simulink model "SkywalkerX8_Lateral_Verification"  (R2018a)
settings: Solver=FixedStepAuto  StartTime=0.0  StopTime=10.0  FixedStep=0.001  RelTol=1e-3
settings Model: Creator=David  LastModifiedBy=David
settings DataIOCC: SaveFormat=StructureWithTime
settings OptimizationCC: BlockReduction=off  BufferReuse=off
settings DebuggingCC: AlgebraicLoopMsg=none  UnconnectedInputMsg=none  UnconnectedOutputMsg=none  UnconnectedLineMsg=none

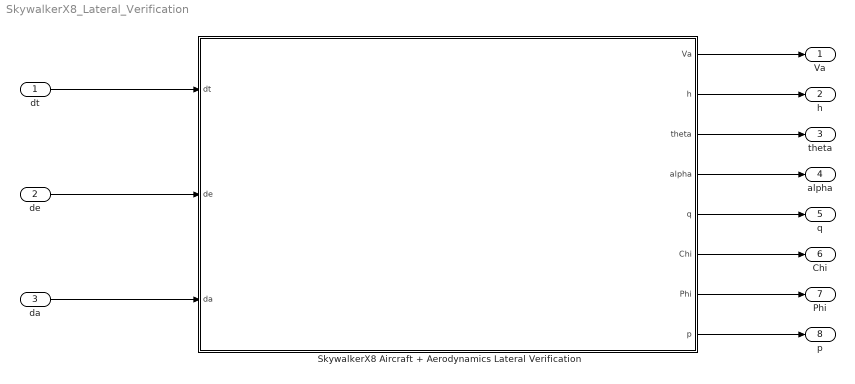
== system SkywalkerX8_Lateral_Verification ==
  dt : Inport
  de : Inport  Port=2
  da : Inport  Port=3
  SkywalkerX8 Aircraft + Aerodynamics Lateral Verification : Subsystem
      mask Display:
      | image('x8SkySunset.png', 'center')
      | 
      | port_label('input', 1, '\delta_t (Unitless)', 'texmode', 'on')
      | port_label('input', 2, '\delta_e (rad)', 'texmode', 'on')
      | port_label('input', 3, '\delta_a (rad)', 'texmode', 'on')
      | 
      | port_label('output', 1, 'V_a (m/s)', 'texmode', 'on')
      | port_label('output', 2, 'Altitude (m)', 'texmode', 'on')
      | port_label('output', 3, '\theta (rad)', 'texmode', 'on')
      | port_label('output', 4, 'alpha (rad)', 'texmode', 'on')
      | port_label('output', 5, 'q (rad/s)', 'texmode', 'on')
      | port_label('output', 6, '\chi (rad)', 'texmode', 'on')
      | port_label('output', 7, '\Phi (rad)', 'texmode', 'on')
      | port_label('output', 8, 'p (rad/s)', 'texmode', 'on')
  Va : Outport
  h : Outport  Port=2
  theta : Outport  Port=3
  alpha : Outport  Port=4
  q : Outport  Port=5
  Chi : Outport  Port=6
  Phi : Outport  Port=7
  p : Outport  Port=8
  wires:
  dt/1 -> SkywalkerX8 Aircraft + Aerodynamics Lateral Verification/1(dt)
  de/1 -> SkywalkerX8 Aircraft + Aerodynamics Lateral Verification/2(de)
  da/1 -> SkywalkerX8 Aircraft + Aerodynamics Lateral Verification/3(da)
  SkywalkerX8 Aircraft + Aerodynamics Lateral Verification/1(Va) -> Va/1
  SkywalkerX8 Aircraft + Aerodynamics Lateral Verification/6(Chi) -> Chi/1
  SkywalkerX8 Aircraft + Aerodynamics Lateral Verification/7(Phi) -> Phi/1
  SkywalkerX8 Aircraft + Aerodynamics Lateral Verification/8(p) -> p/1
  SkywalkerX8 Aircraft + Aerodynamics Lateral Verification/2(h) -> h/1
  SkywalkerX8 Aircraft + Aerodynamics Lateral Verification/3(theta) -> theta/1
  SkywalkerX8 Aircraft + Aerodynamics Lateral Verification/4(alpha) -> alpha/1
  SkywalkerX8 Aircraft + Aerodynamics Lateral Verification/5(q) -> q/1

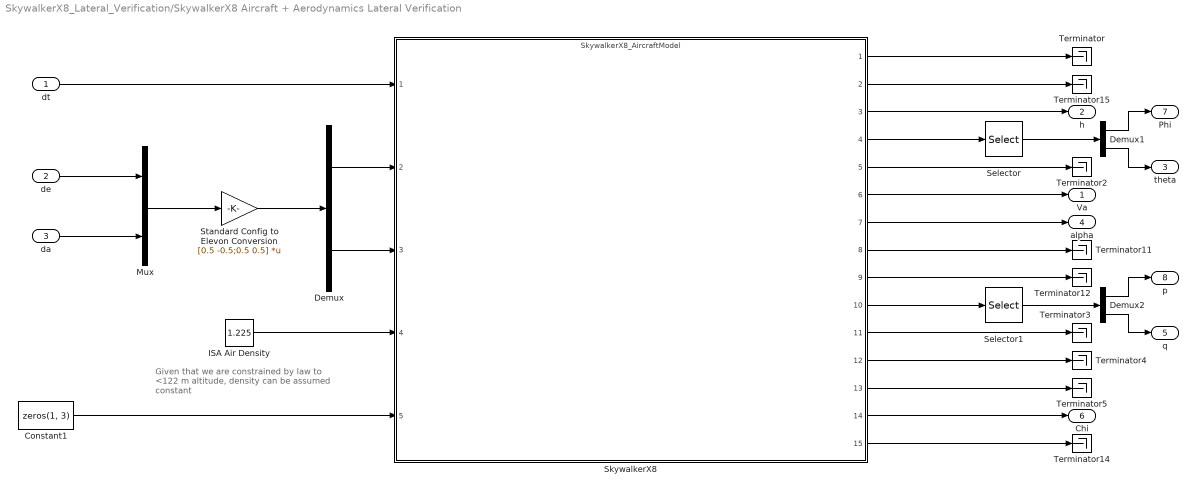
== system SkywalkerX8_Lateral_Verification/SkywalkerX8 Aircraft + Aerodynamics Lateral Verification ==
  note: Given that we are constrained by law to
      | <122 m altitude, density can be assumed
      | constant
  dt : Inport
  de : Inport  Port=2
  da : Inport  Port=3
  Constant1 : Constant  Value=zeros(1, 3)
  Demux : Demux  Outputs=2
  Demux1 : Demux  Outputs=2
  Demux2 : Demux  Outputs=2
  ISA Air Density : Constant  Value=1.225
  Mux : Mux  Inputs=2
  Selector : Selector  InputPortWidth=3  IndexOptions=Index vector (dialog)  Indices=[1, 2]  OutputSizes=1
  Selector1 : Selector  InputPortWidth=3  IndexOptions=Index vector (dialog)  Indices=[1, 2]  OutputSizes=1
  SkywalkerX8 : ModelReference  ModelNameDialog=SkywalkerX8_AircraftModel  ModelReferenceVersion=1.361
      mask Display:
      | image('C:\MATLAB\masters\icons\Skywalker Main Block Icon.png', 'center')
      | 
      | color('cyan')
      | 
      | port_label('input', 1, 'k_{motor} (Unitless)', 'texmode', 'on')
      | port_label('input', 2, '\delta_{er} (rad)', 'texmode', 'on')
      | port_label('input', 3, '\delta_{el} (rad)', 'texmode', 'on')
      | port_label('input', 4, '\rho (kg/m^3)', 'texmode', 'on')
      | port_label('input', 5, '{\bf V_w^b} (m/s)', 'texmode', 'on')
      | 
      | port_label('output', 1, '{\bf V_e} (m/s)', 'texmode', 'on')
      | port_label('output', 2, '{\bf X_e} (m)', 'texmode', 'on')
      | port_label('output', 3, 'Altitude (m)', 'texmode', 'on')
      | port_label('output', 4, '\phi \theta \psi (rad)', 'texmode', 'on')
      | port_label('output', 5, 'R_{inertial}^{body}', 'texmode', 'on')
      | port_label('output', 6, 'V_a (m/s)', 'texmode', 'on')
      | port_label('output', 7, 'alpha (rad)', 'texmode', 'on')
      | port_label('output', 8, 'beta (rad)', 'texmode', 'on')
      | port_label('output', 9, '{\bf V_b} (m/s)', 'texmode', 'on')
      | port_label('output', 10, '{\bf \omega_b} (rad/s)', 'texmode', 'on')
      | port_label('output', 11, '{\bf \delta\omega_b/\deltat} (rad/s^2)', 'texmode', 'on')
      | port_label('output', 12, '{\bf a_{body}} (m/s^2)', 'texmode', 'on')
      | port_label('output', 13, '{\bf a_{inertial}} (m/s^2)', 'texmode', 'on')
      | port_label('output', 14, '\chi (rad)', 'texmode', 'on')
      | port_label('output', 15, '\chi_c (rad)', 'texmode', 'on')
  Standard Config to Elevon Conversion : Gain  Gain=[0.5 -0.5;0.5 0.5]  Multiplication=Matrix(K*u)
  Terminator{,2..5,11..12,14..15} (9 alike) : Terminator
  Va : Outport
  h : Outport  Port=2
  theta : Outport  Port=3
  alpha : Outport  Port=4
  q : Outport  Port=5
  Chi : Outport  Port=6
  Phi : Outport  Port=7
  p : Outport  Port=8
  wires:
  SkywalkerX8/12 -> Terminator4/1
  Demux/2 -> SkywalkerX8/3
  SkywalkerX8/13 -> Terminator5/1
  Mux/1 -> Standard Config to Elevon Conversion/1
  Constant1/1 -> SkywalkerX8/5
  SkywalkerX8/11 -> Terminator3/1
  SkywalkerX8/1 -> Terminator/1
  SkywalkerX8/5 -> Terminator2/1
  Standard Config to Elevon Conversion/1 -> Demux/1
  de/1 -> Mux/1
  Demux/1 -> SkywalkerX8/2
  SkywalkerX8/7 -> alpha/1
  dt/1 -> SkywalkerX8/1
  da/1 -> Mux/2
  SkywalkerX8/8 -> Terminator11/1
  SkywalkerX8/3 -> h/1
  SkywalkerX8/9 -> Terminator12/1
  SkywalkerX8/10 -> Selector1/1
  SkywalkerX8/2 -> Terminator15/1
  SkywalkerX8/4 -> Selector/1
  SkywalkerX8/15 -> Terminator14/1
  ISA Air Density/1 -> SkywalkerX8/4
  SkywalkerX8/14 -> Chi/1
  SkywalkerX8/6 -> Va/1
  Selector/1 -> Demux1/1
  Demux1/1 -> Phi/1
  Demux1/2 -> theta/1
  Selector1/1 -> Demux2/1
  Demux2/1 -> p/1
  Demux2/2 -> q/1
